simulink model "IEEE9_case"  (R2024b)
settings: Solver=FixedStepAuto  StartTime=0  StopTime=5  FixedStep=1e-7  RelTol=1e-3
values from neighbouring files (symbols this model uses):
  SG_D_1_D = 0.01056    [IEEE9_case_parameters.m]    (also in case1_parameters.m; case2_parameters.m; case3_parameters.m; case4_parameters.m)
  SG_D_1_EnableSaturation = 0    [IEEE9_case_parameters.m]    (also in case1_parameters.m; case2_parameters.m; case3_parameters.m; case4_parameters.m)
  SG_D_1_f0 = 60    [IEEE9_case_parameters.m]    (also in case1_parameters.m; case2_parameters.m; case3_parameters.m; case4_parameters.m)
  SG_D_1_H = 7.5    [IEEE9_case_parameters.m]    (also in case1_parameters.m; case2_parameters.m; case3_parameters.m; case4_parameters.m)
  SG_D_1_K_A = 20    [IEEE9_case_parameters.m]    (also in case1_parameters.m; case2_parameters.m; case3_parameters.m; case4_parameters.m)
  SG_D_1_K_E = 1.000000e+1    (= 10)    [IEEE9_case_parameters.m]    (also in case1_parameters.m; case2_parameters.m; case3_parameters.m; case4_parameters.m)
  SG_D_1_K_F = 2.363    [IEEE9_case_parameters.m]    (also in case1_parameters.m; case2_parameters.m; case3_parameters.m; case4_parameters.m)
  SG_D_1_K_s = 0.5    [IEEE9_case_parameters.m]    (also in case1_parameters.m = 5; case2_parameters.m = 5; case3_parameters.m = 5; case4_parameters.m = 5)
  SG_D_1_R_a = 0.001088    [IEEE9_case_parameters.m]    (also in case1_parameters.m; case2_parameters.m; case3_parameters.m; case4_parameters.m)
  SG_D_1_S_A = 1    [IEEE9_case_parameters.m]    (also in case1_parameters.m; case2_parameters.m; case3_parameters.m; case4_parameters.m)
  SG_D_1_S_B = 0.103    [IEEE9_case_parameters.m]    (also in case1_parameters.m; case2_parameters.m; case3_parameters.m; case4_parameters.m)
  SG_D_1_S_N = 10.659857    [IEEE9_case_parameters.m]    (also in case1_parameters.m; case2_parameters.m; case3_parameters.m; case4_parameters.m)
  SG_D_1_SpeedPara = 200    [IEEE9_case_parameters.m]    (also in case1_parameters.m; case2_parameters.m; case3_parameters.m; case4_parameters.m)
  SG_D_1_T_0 = 0.720173    [IEEE9_case_parameters.m]    (also in case1_parameters.m = 0.755522; case2_parameters.m = 0.808931; case3_parameters.m = 0.869402; case4_parameters.m = 0.729316)
  SG_D_1_T_1 = 0.3    [IEEE9_case_parameters.m]    (also in case1_parameters.m; case2_parameters.m; case3_parameters.m; case4_parameters.m)
  SG_D_1_T_2 = 0.05    [IEEE9_case_parameters.m]    (also in case1_parameters.m; case2_parameters.m; case3_parameters.m; case4_parameters.m)
  SG_D_1_T_3 = 0.02    [IEEE9_case_parameters.m]    (also in case1_parameters.m; case2_parameters.m; case3_parameters.m; case4_parameters.m)
  SG_D_1_T_4 = 0.005    [IEEE9_case_parameters.m]    (also in case1_parameters.m; case2_parameters.m; case3_parameters.m; case4_parameters.m)
  SG_D_1_T_A = 0.02    [IEEE9_case_parameters.m]    (also in case1_parameters.m; case2_parameters.m; case3_parameters.m; case4_parameters.m)
  SG_D_1_T_dd = 8.000000e+0    (= 8)    [IEEE9_case_parameters.m]    (also in case1_parameters.m; case2_parameters.m; case3_parameters.m; case4_parameters.m)
  SG_D_1_T_ddd = 0.04    [IEEE9_case_parameters.m]    (also in case1_parameters.m; case2_parameters.m; case3_parameters.m; case4_parameters.m)
  SG_D_1_T_E = 0.314    [IEEE9_case_parameters.m]    (also in case1_parameters.m; case2_parameters.m; case3_parameters.m; case4_parameters.m)
  SG_D_1_T_F = 0.35    [IEEE9_case_parameters.m]    (also in case1_parameters.m; case2_parameters.m; case3_parameters.m; case4_parameters.m)
  SG_D_1_T_qd = 0.8    [IEEE9_case_parameters.m]    (also in case1_parameters.m; case2_parameters.m; case3_parameters.m; case4_parameters.m)
  SG_D_1_T_qdd = 0.02    [IEEE9_case_parameters.m]    (also in case1_parameters.m; case2_parameters.m; case3_parameters.m; case4_parameters.m)
  SG_D_1_T_speed = 0.1    [IEEE9_case_parameters.m]    (also in case1_parameters.m = 200; case2_parameters.m = 200; case3_parameters.m = 200; case4_parameters.m = 200)
  SG_D_1_T_w = 0.5    [IEEE9_case_parameters.m]    (also in case1_parameters.m; case2_parameters.m; case3_parameters.m; case4_parameters.m)
  SG_D_1_V_ref = 1.990276    [IEEE9_case_parameters.m]    (also in case1_parameters.m = 2.042296; case2_parameters.m = 2.051388; case3_parameters.m = 2.089584; case4_parameters.m = 2.01845)
  SG_D_1_w_ref = 376.991118    [IEEE9_case_parameters.m]    (also in case1_parameters.m; case2_parameters.m; case3_parameters.m; case4_parameters.m)
  SG_D_1_wb = 6.000000e+1    (= 60)    [IEEE9_case_parameters.m]    (also in case1_parameters.m; case2_parameters.m; case3_parameters.m; case4_parameters.m)
  SG_D_1_x_d = 1.9    [IEEE9_case_parameters.m]    (also in case1_parameters.m; case2_parameters.m; case3_parameters.m; case4_parameters.m)
  SG_D_1_x_dd = 0.302    [IEEE9_case_parameters.m]    (also in case1_parameters.m; case2_parameters.m; case3_parameters.m; case4_parameters.m)
  SG_D_1_x_ddd = 0.204    [IEEE9_case_parameters.m]    (also in case1_parameters.m; case2_parameters.m; case3_parameters.m; case4_parameters.m)
  SG_D_1_x_l = 0.05    [IEEE9_case_parameters.m]    (also in case1_parameters.m; case2_parameters.m; case3_parameters.m; case4_parameters.m)
  SG_D_1_x_q = 1.3    [IEEE9_case_parameters.m]    (also in case1_parameters.m; case2_parameters.m; case3_parameters.m; case4_parameters.m)
  SG_D_1_x_qd = 0.5    [IEEE9_case_parameters.m]    (also in case1_parameters.m; case2_parameters.m; case3_parameters.m; case4_parameters.m)
  SG_D_1_x_qdd = 0.3    [IEEE9_case_parameters.m]    (also in case1_parameters.m; case2_parameters.m; case3_parameters.m; case4_parameters.m)
  SG_D_2_D = 0.02    [IEEE9_case_parameters.m]    (also in case1_parameters.m; case2_parameters.m; case3_parameters.m; case4_parameters.m)
  SG_D_2_EnableSaturation = 0    [IEEE9_case_parameters.m]    (also in case1_parameters.m; case2_parameters.m; case3_parameters.m; case4_parameters.m)
  SG_D_2_f0 = 60    [IEEE9_case_parameters.m]    (also in case1_parameters.m; case2_parameters.m; case3_parameters.m; case4_parameters.m)
  SG_D_2_H = 8.000000e+0    (= 8)    [IEEE9_case_parameters.m]    (also in case1_parameters.m; case2_parameters.m; case3_parameters.m; case4_parameters.m)
  SG_D_2_K_A = 20    [IEEE9_case_parameters.m]    (also in case1_parameters.m; case2_parameters.m; case3_parameters.m; case4_parameters.m)
  SG_D_2_K_E = 1.000000e+1    (= 10)    [IEEE9_case_parameters.m]    (also in case1_parameters.m; case2_parameters.m; case3_parameters.m; case4_parameters.m)
  SG_D_2_K_F = 2.363    [IEEE9_case_parameters.m]    (also in case1_parameters.m; case2_parameters.m; case3_parameters.m; case4_parameters.m)
  SG_D_2_K_s = 0.5    [IEEE9_case_parameters.m]    (also in case1_parameters.m = 4; case2_parameters.m = 4; case3_parameters.m = 4; case4_parameters.m = 4)
  SG_D_2_R_a = 0.001088    [IEEE9_case_parameters.m]    (also in case1_parameters.m; case2_parameters.m; case3_parameters.m; case4_parameters.m)
  SG_D_2_S_A = 1    [IEEE9_case_parameters.m]    (also in case1_parameters.m; case2_parameters.m; case3_parameters.m; case4_parameters.m)
  SG_D_2_S_B = 0.103    [IEEE9_case_parameters.m]    (also in case1_parameters.m; case2_parameters.m; case3_parameters.m; case4_parameters.m)
  SG_D_2_S_N = 10.659857    [IEEE9_case_parameters.m]    (also in case1_parameters.m; case2_parameters.m; case3_parameters.m; case4_parameters.m)
  SG_D_2_SpeedPara = 200    [IEEE9_case_parameters.m]    (also in case1_parameters.m; case2_parameters.m; case3_parameters.m; case4_parameters.m)
  SG_D_2_T_0 = 1.632913    [IEEE9_case_parameters.m]    (also in case1_parameters.m = 1.632925; case2_parameters.m = 1.632915; case3_parameters.m = 1.632914; case4_parameters.m = 1.632927)
  SG_D_2_T_1 = 0.2    [IEEE9_case_parameters.m]    (also in case1_parameters.m; case2_parameters.m; case3_parameters.m; case4_parameters.m)
  SG_D_2_T_2 = 0.05    [IEEE9_case_parameters.m]    (also in case1_parameters.m; case2_parameters.m; case3_parameters.m; case4_parameters.m)
  SG_D_2_T_3 = 0.02    [IEEE9_case_parameters.m]    (also in case1_parameters.m; case2_parameters.m; case3_parameters.m; case4_parameters.m)
  SG_D_2_T_4 = 0.005    [IEEE9_case_parameters.m]    (also in case1_parameters.m; case2_parameters.m; case3_parameters.m; case4_parameters.m)
  SG_D_2_T_A = 0.02    [IEEE9_case_parameters.m]    (also in case1_parameters.m; case2_parameters.m; case3_parameters.m; case4_parameters.m)
  SG_D_2_T_dd = 7.9    [IEEE9_case_parameters.m]    (also in case1_parameters.m; case2_parameters.m; case3_parameters.m; case4_parameters.m)
  SG_D_2_T_ddd = 0.04    [IEEE9_case_parameters.m]    (also in case1_parameters.m; case2_parameters.m; case3_parameters.m; case4_parameters.m)
  SG_D_2_T_E = 0.314    [IEEE9_case_parameters.m]    (also in case1_parameters.m; case2_parameters.m; case3_parameters.m; case4_parameters.m)
  SG_D_2_T_F = 0.35    [IEEE9_case_parameters.m]    (also in case1_parameters.m; case2_parameters.m; case3_parameters.m; case4_parameters.m)
  SG_D_2_T_qd = 0.8    [IEEE9_case_parameters.m]    (also in case1_parameters.m; case2_parameters.m; case3_parameters.m; case4_parameters.m)
  SG_D_2_T_qdd = 0.015    [IEEE9_case_parameters.m]    (also in case1_parameters.m; case2_parameters.m; case3_parameters.m; case4_parameters.m)
  SG_D_2_T_speed = 0.1    [IEEE9_case_parameters.m]    (also in case1_parameters.m = 150; case2_parameters.m = 150; case3_parameters.m = 150; case4_parameters.m = 150)
  SG_D_2_T_w = 0.35    [IEEE9_case_parameters.m]    (also in case1_parameters.m; case2_parameters.m; case3_parameters.m; case4_parameters.m)
  SG_D_2_V_ref = 2.58547    [IEEE9_case_parameters.m]    (also in case1_parameters.m = 2.597896; case2_parameters.m = 2.587136; case3_parameters.m = 2.586042; case4_parameters.m = 2.599679)
  SG_D_2_w_ref = 376.991118    [IEEE9_case_parameters.m]    (also in case1_parameters.m; case2_parameters.m; case3_parameters.m; case4_parameters.m)
  SG_D_2_wb = 6.000000e+1    (= 60)    [IEEE9_case_parameters.m]    (also in case1_parameters.m; case2_parameters.m; case3_parameters.m; case4_parameters.m)
  SG_D_2_x_d = 1.8    [IEEE9_case_parameters.m]    (also in case1_parameters.m; case2_parameters.m; case3_parameters.m; case4_parameters.m)
  SG_D_2_x_dd = 0.302    [IEEE9_case_parameters.m]    (also in case1_parameters.m; case2_parameters.m; case3_parameters.m; case4_parameters.m)
  SG_D_2_x_ddd = 0.204    [IEEE9_case_parameters.m]    (also in case1_parameters.m; case2_parameters.m; case3_parameters.m; case4_parameters.m)
  SG_D_2_x_l = 0.05    [IEEE9_case_parameters.m]    (also in case1_parameters.m; case2_parameters.m; case3_parameters.m; case4_parameters.m)
  SG_D_2_x_q = 1.25    [IEEE9_case_parameters.m]    (also in case1_parameters.m; case2_parameters.m; case3_parameters.m; case4_parameters.m)
  SG_D_2_x_qd = 0.5    [IEEE9_case_parameters.m]    (also in case1_parameters.m; case2_parameters.m; case3_parameters.m; case4_parameters.m)
  SG_D_2_x_qdd = 0.3    [IEEE9_case_parameters.m]    (also in case1_parameters.m; case2_parameters.m; case3_parameters.m; case4_parameters.m)
  SG_D_3_D = 0.02    [IEEE9_case_parameters.m]    (also in case1_parameters.m; case2_parameters.m; case3_parameters.m; case4_parameters.m)
  SG_D_3_EnableSaturation = 0    [IEEE9_case_parameters.m]    (also in case1_parameters.m; case2_parameters.m; case3_parameters.m; case4_parameters.m)
  SG_D_3_f0 = 60    [IEEE9_case_parameters.m]    (also in case1_parameters.m; case2_parameters.m; case3_parameters.m; case4_parameters.m)
  SG_D_3_H = 7.7    [IEEE9_case_parameters.m]    (also in case1_parameters.m; case2_parameters.m; case3_parameters.m; case4_parameters.m)
  SG_D_3_K_A = 20    [IEEE9_case_parameters.m]    (also in case1_parameters.m; case2_parameters.m; case3_parameters.m; case4_parameters.m)
  SG_D_3_K_E = 1.000000e+1    (= 10)    [IEEE9_case_parameters.m]    (also in case1_parameters.m; case2_parameters.m; case3_parameters.m; case4_parameters.m)
  SG_D_3_K_F = 2.363    [IEEE9_case_parameters.m]    (also in case1_parameters.m; case2_parameters.m; case3_parameters.m; case4_parameters.m)
  SG_D_3_K_s = 0.2    [IEEE9_case_parameters.m]    (also in case1_parameters.m = 2; case2_parameters.m = 2; case3_parameters.m = 2; case4_parameters.m = 2)
  SG_D_3_R_a = 0.001088    [IEEE9_case_parameters.m]    (also in case1_parameters.m; case2_parameters.m; case3_parameters.m; case4_parameters.m)
  SG_D_3_S_A = 1    [IEEE9_case_parameters.m]    (also in case1_parameters.m; case2_parameters.m; case3_parameters.m; case4_parameters.m)
  SG_D_3_S_B = 0.103    [IEEE9_case_parameters.m]    (also in case1_parameters.m; case2_parameters.m; case3_parameters.m; case4_parameters.m)
  SG_D_3_S_N = 10.659857    [IEEE9_case_parameters.m]    (also in case1_parameters.m; case2_parameters.m; case3_parameters.m; case4_parameters.m)
  SG_D_3_SpeedPara = 200    [IEEE9_case_parameters.m]    (also in case1_parameters.m; case2_parameters.m; case3_parameters.m; case4_parameters.m)
  SG_D_3_T_0 = 0.850788    [IEEE9_case_parameters.m]    (also in case1_parameters.m = 0.850786; case2_parameters.m = 0.850787; case3_parameters.m; case4_parameters.m = 0.850786)
  SG_D_3_T_1 = 0.2    [IEEE9_case_parameters.m]    (also in case1_parameters.m; case2_parameters.m; case3_parameters.m; case4_parameters.m)
  SG_D_3_T_2 = 0.05    [IEEE9_case_parameters.m]    (also in case1_parameters.m; case2_parameters.m; case3_parameters.m; case4_parameters.m)
  SG_D_3_T_3 = 0.02    [IEEE9_case_parameters.m]    (also in case1_parameters.m; case2_parameters.m; case3_parameters.m; case4_parameters.m)
  SG_D_3_T_4 = 0.005    [IEEE9_case_parameters.m]    (also in case1_parameters.m; case2_parameters.m; case3_parameters.m; case4_parameters.m)
  SG_D_3_T_A = 0.02    [IEEE9_case_parameters.m]    (also in case1_parameters.m; case2_parameters.m; case3_parameters.m; case4_parameters.m)
  SG_D_3_T_dd = 8.1    [IEEE9_case_parameters.m]    (also in case1_parameters.m; case2_parameters.m; case3_parameters.m; case4_parameters.m)
  SG_D_3_T_ddd = 0.04    [IEEE9_case_parameters.m]    (also in case1_parameters.m; case2_parameters.m; case3_parameters.m; case4_parameters.m)
  SG_D_3_T_E = 0.314    [IEEE9_case_parameters.m]    (also in case1_parameters.m; case2_parameters.m; case3_parameters.m; case4_parameters.m)
  SG_D_3_T_F = 0.35    [IEEE9_case_parameters.m]    (also in case1_parameters.m; case2_parameters.m; case3_parameters.m; case4_parameters.m)
  SG_D_3_T_qd = 0.8    [IEEE9_case_parameters.m]    (also in case1_parameters.m; case2_parameters.m; case3_parameters.m; case4_parameters.m)
  SG_D_3_T_qdd = 0.015    [IEEE9_case_parameters.m]    (also in case1_parameters.m; case2_parameters.m; case3_parameters.m; case4_parameters.m)
  SG_D_3_T_speed = 0.1    [IEEE9_case_parameters.m]    (also in case1_parameters.m = 180; case2_parameters.m = 180; case3_parameters.m = 180; case4_parameters.m = 180)
  SG_D_3_T_w = 0.4    [IEEE9_case_parameters.m]    (also in case1_parameters.m; case2_parameters.m; case3_parameters.m; case4_parameters.m)
  SG_D_3_V_ref = 1.892727    [IEEE9_case_parameters.m]    (also in case1_parameters.m = 1.906439; case2_parameters.m = 1.895535; case3_parameters.m = 1.892105; case4_parameters.m = 1.906598)
  SG_D_3_w_ref = 376.991118    [IEEE9_case_parameters.m]    (also in case1_parameters.m; case2_parameters.m; case3_parameters.m; case4_parameters.m)
  SG_D_3_wb = 6.000000e+1    (= 60)    [IEEE9_case_parameters.m]    (also in case1_parameters.m; case2_parameters.m; case3_parameters.m; case4_parameters.m)
  SG_D_3_x_d = 1.85    [IEEE9_case_parameters.m]    (also in case1_parameters.m; case2_parameters.m; case3_parameters.m; case4_parameters.m)
  SG_D_3_x_dd = 0.302    [IEEE9_case_parameters.m]    (also in case1_parameters.m; case2_parameters.m; case3_parameters.m; case4_parameters.m)
  SG_D_3_x_ddd = 0.204    [IEEE9_case_parameters.m]    (also in case1_parameters.m; case2_parameters.m; case3_parameters.m; case4_parameters.m)
  SG_D_3_x_l = 0.05    [IEEE9_case_parameters.m]    (also in case1_parameters.m; case2_parameters.m; case3_parameters.m; case4_parameters.m)
  SG_D_3_x_q = 1.2    [IEEE9_case_parameters.m]    (also in case1_parameters.m; case2_parameters.m; case3_parameters.m; case4_parameters.m)
  SG_D_3_x_qd = 0.5    [IEEE9_case_parameters.m]    (also in case1_parameters.m; case2_parameters.m; case3_parameters.m; case4_parameters.m)
  SG_D_3_x_qdd = 0.3    [IEEE9_case_parameters.m]    (also in case1_parameters.m; case2_parameters.m; case3_parameters.m; case4_parameters.m)
(part 9 of 12)

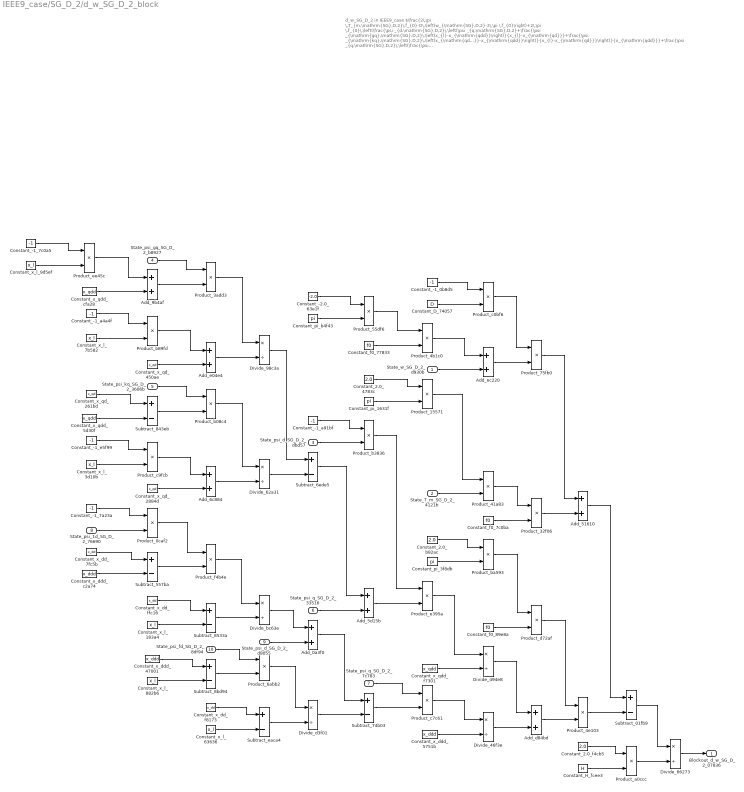
== system IEEE9_case/SG_D_2/d_w_SG_D_2_block ==
  note: d_w_SG_D_2 in IEEE9_case
      | $\frac{2\,\pi \,T_{m,\mathrm{SG},D,2}\,f_{0}-D\,\left(w_{\mathrm{SG},D,2}-2\,\pi \,f_{0}\right)+2\,\pi \,f_{0}\,\left(\frac{\psi _{d,\mathrm{SG},D,2}\,\left(\psi _{q,\mathrm{SG},D,2}+\frac{\psi _{\mathrm{gq},\mathrm{SG},D,2}\,\left(x_{l}-x_{\mathrm{qdd}}\right)}{x_{l}-x_{\mathrm{qd}}}+\frac{\psi _{\mathrm{kq},\mathrm{SG},D,2}\,\left(x_{\mathrm{qd}}-x_{\mathrm{qdd}}\right)}{x_{l}-x_{\mathrm{qd}}}\right)}{x_{\mathrm{qdd}}}+\frac{\psi _{q,\mathrm{SG},D,2}\,\left(\frac{\psi _{\mathrm{1d},\mathrm{SG},D,2}\,\left(x_{\mathrm{dd}}-x_{\mathrm{ddd}}\right)}{x_{\mathrm{dd}}-x_{l}}-\psi _{d,\mathrm{SG},D,2}+\frac{\psi _{\mathrm{fd},\mathrm{SG},D,2}\,\left(x_{\mathrm{ddd}}-x_{l}\right)}{x_{\mathrm{dd}}-x_{l}}\right)}{x_{\mathrm{ddd}}}\right)}{2\,H}$
      | Automatically generated on 2025-11-01 08:48:58 .
  State_w_SG_D_2_d930b : Inport
  State_T_m_SG_D_2_4121b : Inport  Port=2
  State_psi_d_SG_D_2_dbd57 : Inport  Port=3
  State_psi_gq_SG_D_2_b8927 : Inport  Port=4
  State_psi_kq_SG_D_2_3606b : Inport  Port=5
  State_psi_q_SG_D_2_33516 : Inport  Port=6
  State_psi_q_SG_D_2_7c783 : Inport  Port=7
  State_psi_1d_SG_D_2_76690 : Inport  Port=8
  State_psi_d_SG_D_2_d8055 : Inport  Port=9
  State_psi_fd_SG_D_2_8df94 : Inport  Port=10
  Add_0a3f0 : Sum
  Add_51610 : Sum
  Add_5d15b : Sum
  Add_6c884 : Sum
  Add_9b4af : Sum
  Add_d84bd : Sum
  Add_e04e4 : Sum
  Add_ec220 : Sum
  Constant_-1_0b8d5 : Constant  Value=-1
  Constant_-1_7a23a : Constant  Value=-1
  Constant_-1_7c0a5 : Constant  Value=-1
  Constant_-1_a4a4f : Constant  Value=-1
  Constant_-1_a91bf : Constant  Value=-1
  Constant_-1_e5f99 : Constant  Value=-1
  Constant_-2.0_63e1f : Constant  Value=-2.0
  Constant_2.0_4783c : Constant  Value=2.0
  Constant_2.0_b82ac : Constant  Value=2.0
  Constant_2.0_f4cb5 : Constant  Value=2.0
  Constant_D_74057 : Constant  Value=D
  Constant_H_fcee3 : Constant  Value=H
  Constant_f0_77833 : Constant  Value=f0
  Constant_f0_7c0ba : Constant  Value=f0
  Constant_f0_89e8a : Constant  Value=f0
  Constant_pi_1631f : Constant  Value=pi
  Constant_pi_3f8db : Constant  Value=pi
  Constant_pi_b4f43 : Constant  Value=pi
  Constant_x_dd_7fc5b : Constant  Value=x_dd
  Constant_x_dd_f8173 : Constant  Value=x_dd
  Constant_x_dd_ffc16 : Constant  Value=x_dd
  Constant_x_ddd_47001 : Constant  Value=x_ddd
  Constant_x_ddd_5751b : Constant  Value=x_ddd
  Constant_x_ddd_c2a74 : Constant  Value=x_ddd
  Constant_x_l_183a4 : Constant  Value=x_l
  Constant_x_l_3d10b : Constant  Value=x_l
  Constant_x_l_63636 : Constant  Value=x_l
  Constant_x_l_7b582 : Constant  Value=x_l
  Constant_x_l_882b6 : Constant  Value=x_l
  Constant_x_l_9d5ef : Constant  Value=x_l
  Constant_x_qd_261bd : Constant  Value=x_qd
  Constant_x_qd_2884d : Constant  Value=x_qd
  Constant_x_qd_450ae : Constant  Value=x_qd
  Constant_x_qdd_5d30f : Constant  Value=x_qdd
  Constant_x_qdd_cfa28 : Constant  Value=x_qdd
  Constant_x_qdd_f7301 : Constant  Value=x_qdd
  Divide_46f3e : Product  Inputs=*/
  Divide_494e8 : Product  Inputs=*/
  Divide_62a31 : Product  Inputs=*/
  Divide_66273 : Product  Inputs=*/
  Divide_98c3a : Product  Inputs=*/
  Divide_bc63e : Product  Inputs=*/
  Divide_d3f01 : Product  Inputs=*/
  Product_0caf2 : Product
  Product_15571 : Product
  Product_32f06 : Product
  Product_3add3 : Product
  Product_41a83 : Product
  Product_4b1c0 : Product
  Product_4e103 : Product
  Product_55df6 : Product
  Product_6abb2 : Product
  Product_75fb0 : Product
  Product_a0ccc : Product
  Product_b08c4 : Product
  Product_b3836 : Product
  Product_b89fd : Product
  Product_ba593 : Product
  Product_c0bf6 : Product
  Product_c7c61 : Product
  Product_c9fcb : Product
  Product_d72af : Product
  Product_e395a : Product
  Product_ee45c : Product
  Product_f4b4e : Product
  Subtract_01fb9 : Sum  Inputs=+-
  Subtract_557ba : Sum  Inputs=+-
  Subtract_6ede5 : Sum  Inputs=+-
  Subtract_74b03 : Sum  Inputs=+-
  Subtract_843eb : Sum  Inputs=+-
  Subtract_8533a : Sum  Inputs=+-
  Subtract_8bd94 : Sum  Inputs=+-
  Subtract_eaca4 : Sum  Inputs=+-
  Blockout_d_w_SG_D_2_07836 : Outport
  wires:
  Constant_x_qd_261bd/1 -> Subtract_843eb/1
  Constant_-1_e5f99/1 -> Product_c9fcb/1
  Constant_-1_7c0a5/1 -> Product_ee45c/1
  Constant_x_qdd_5d30f/1 -> Subtract_843eb/2
  Subtract_eaca4/1 -> Divide_d3f01/2
  Constant_x_l_3d10b/1 -> Product_c9fcb/2
  Constant_x_l_9d5ef/1 -> Product_ee45c/2
  Product_c9fcb/1 -> Add_6c884/1
  Product_ee45c/1 -> Add_9b4af/1
  Constant_x_l_183a4/1 -> Subtract_8533a/2
  Constant_x_l_7b582/1 -> Product_b89fd/2
  Constant_x_ddd_5751b/1 -> Divide_46f3e/2
  Subtract_8bd94/1 -> Product_6abb2/2
  Constant_x_qd_2884d/1 -> Add_6c884/2
  Constant_x_qdd_cfa28/1 -> Add_9b4af/2
  Constant_-1_a4a4f/1 -> Product_b89fd/1
  State_psi_d_SG_D_2_dbd57/1 -> Product_b3836/2
  Constant_-1_7a23a/1 -> Product_0caf2/1
  State_w_SG_D_2_d930b/1 -> Add_ec220/2
  Product_b89fd/1 -> Add_e04e4/1
  State_psi_1d_SG_D_2_76690/1 -> Product_0caf2/2
  Constant_x_dd_7fc5b/1 -> Subtract_557ba/1
  Divide_98c3a/1 -> Subtract_6ede5/1
  Subtract_843eb/1 -> Product_b08c4/2
  Constant_x_ddd_c2a74/1 -> Subtract_557ba/2
  State_psi_gq_SG_D_2_b8927/1 -> Product_3add3/1
  Add_6c884/1 -> Divide_62a31/2
  State_psi_d_SG_D_2_d8055/1 -> Add_0a3f0/2
  Add_9b4af/1 -> Product_3add3/2
  Constant_x_qd_450ae/1 -> Add_e04e4/2
  State_psi_kq_SG_D_2_3606b/1 -> Product_b08c4/1
  Product_0caf2/1 -> Product_f4b4e/1
  Subtract_557ba/1 -> Product_f4b4e/2
  Constant_pi_1631f/1 -> Product_15571/2
  Constant_x_dd_ffc16/1 -> Subtract_8533a/1
  Constant_x_ddd_47001/1 -> Subtract_8bd94/1
  Constant_x_l_882b6/1 -> Subtract_8bd94/2
  Product_3add3/1 -> Divide_98c3a/1
  Add_e04e4/1 -> Divide_98c3a/2
  Add_5d15b/1 -> Product_e395a/2
  Product_b08c4/1 -> Divide_62a31/1
  Constant_pi_b4f43/1 -> Product_55df6/2
  Product_f4b4e/1 -> Divide_bc63e/1
  Subtract_8533a/1 -> Divide_bc63e/2
  State_psi_fd_SG_D_2_8df94/1 -> Product_6abb2/1
  Divide_bc63e/1 -> Add_0a3f0/1
  Constant_x_dd_f8173/1 -> Subtract_eaca4/1
  Constant_x_l_63636/1 -> Subtract_eaca4/2
  Divide_62a31/1 -> Subtract_6ede5/2
  Product_6abb2/1 -> Divide_d3f01/1
  Constant_-1_a91bf/1 -> Product_b3836/1
  Constant_-2.0_63e1f/1 -> Product_55df6/1
  Subtract_6ede5/1 -> Add_5d15b/1
  Subtract_74b03/1 -> Product_c7c61/2
  State_psi_q_SG_D_2_33516/1 -> Add_5d15b/2
  Constant_D_74057/1 -> Product_c0bf6/2
  Add_0a3f0/1 -> Subtract_74b03/1
  Divide_d3f01/1 -> Subtract_74b03/2
  Product_55df6/1 -> Product_4b1c0/1
  Constant_f0_77833/1 -> Product_4b1c0/2
  Constant_2.0_4783c/1 -> Product_15571/1
  Product_b3836/1 -> Product_e395a/1
  State_psi_q_SG_D_2_7c783/1 -> Product_c7c61/1
  Constant_-1_0b8d5/1 -> Product_c0bf6/1
  Product_4b1c0/1 -> Add_ec220/1
  Product_15571/1 -> Product_41a83/1
  State_T_m_SG_D_2_4121b/1 -> Product_41a83/2
  Constant_2.0_b82ac/1 -> Product_ba593/1
  Constant_pi_3f8db/1 -> Product_ba593/2
  Product_e395a/1 -> Divide_494e8/1
  Constant_x_qdd_f7301/1 -> Divide_494e8/2
  Product_c7c61/1 -> Divide_46f3e/1
  Product_c0bf6/1 -> Product_75fb0/1
  Add_ec220/1 -> Product_75fb0/2
  Product_41a83/1 -> Product_32f06/1
  Constant_f0_7c0ba/1 -> Product_32f06/2
  Product_ba593/1 -> Product_d72af/1
  Constant_f0_89e8a/1 -> Product_d72af/2
  Divide_494e8/1 -> Add_d84bd/1
  Divide_46f3e/1 -> Add_d84bd/2
  Product_75fb0/1 -> Add_51610/1
  Product_32f06/1 -> Add_51610/2
  Product_d72af/1 -> Product_4e103/1
  Add_d84bd/1 -> Product_4e103/2
  Add_51610/1 -> Subtract_01fb9/1
  Product_4e103/1 -> Subtract_01fb9/2
  Constant_2.0_f4cb5/1 -> Product_a0ccc/1
  Constant_H_fcee3/1 -> Product_a0ccc/2
  Subtract_01fb9/1 -> Divide_66273/1
  Product_a0ccc/1 -> Divide_66273/2
  Divide_66273/1 -> Blockout_d_w_SG_D_2_07836/1

== system IEEE9_case/SG_D_2/i_d_SG_D_2_block ==
  note: i_d_SG_D_2 in IEEE9_case
      | $\frac{\sin\left(\theta _{\mathrm{SG},D,2}\right)\,\left(\frac{\psi _{\mathrm{1d},\mathrm{SG},D,2}\,\left(x_{\mathrm{dd}}-x_{\mathrm{ddd}}\right)}{x_{\mathrm{dd}}-x_{l}}-\psi _{d,\mathrm{SG},D,2}+\frac{\psi _{\mathrm{fd},\mathrm{SG},D,2}\,\left(x_{\mathrm{ddd}}-x_{l}\right)}{x_{\mathrm{dd}}-x_{l}}\right)}{x_{\mathrm{ddd}}}-\frac{\cos\left(\theta _{\mathrm{SG},D,2}\right)\,\left(\psi _{q,\mathrm{SG},D,2}+\frac{\psi _{\mathrm{gq},\mathrm{SG},D,2}\,\left(x_{l}-x_{\mathrm{qdd}}\right)}{x_{l}-x_{\mathrm{qd}}}+\frac{\psi _{\mathrm{kq},\mathrm{SG},D,2}\,\left(x_{\mathrm{qd}}-x_{\mathrm{qdd}}\right)}{x_{l}-x_{\mathrm{qd}}}\right)}{x_{\mathrm{qdd}}}$
      | Automatically generated on 2025-11-01 08:49:20 .
  State_psi_gq_SG_D_2_c758c : Inport
  State_psi_kq_SG_D_2_22efa : Inport  Port=2
  State_psi_q_SG_D_2_90cca : Inport  Port=3
  State_theta_SG_D_2_b69be : Inport  Port=4
  State_psi_1d_SG_D_2_5d51d : Inport  Port=5
  State_psi_d_SG_D_2_f7721 : Inport  Port=6
  State_psi_fd_SG_D_2_83be3 : Inport  Port=7
  State_theta_SG_D_2_1b926 : Inport  Port=8
  Add_16b33 : Sum
  Add_2a93c : Sum
  Add_7d69f : Sum
  Add_a40ae : Sum
  Add_b9970 : Sum
  Constant_-1_8a7ae : Constant  Value=-1
  Constant_-1_a0e83 : Constant  Value=-1
  Constant_-1_cca40 : Constant  Value=-1
  Constant_-1_e0227 : Constant  Value=-1
  Constant_-1_f6edc : Constant  Value=-1
  Constant_x_dd_486e3 : Constant  Value=x_dd
  Constant_x_dd_9e9c9 : Constant  Value=x_dd
  Constant_x_dd_f4509 : Constant  Value=x_dd
  Constant_x_ddd_62481 : Constant  Value=x_ddd
  Constant_x_ddd_8778a : Constant  Value=x_ddd
  Constant_x_ddd_cb7be : Constant  Value=x_ddd
  Constant_x_l_225f2 : Constant  Value=x_l
  Constant_x_l_3670c : Constant  Value=x_l
  Constant_x_l_5d8a7 : Constant  Value=x_l
  Constant_x_l_7740d : Constant  Value=x_l
  Constant_x_l_c677c : Constant  Value=x_l
  Constant_x_l_cd01c : Constant  Value=x_l
  Constant_x_qd_0d99f : Constant  Value=x_qd
  Constant_x_qd_c1993 : Constant  Value=x_qd
  Constant_x_qd_dd2b1 : Constant  Value=x_qd
  Constant_x_qdd_63b5a : Constant  Value=x_qdd
  Constant_x_qdd_7c187 : Constant  Value=x_qdd
  Constant_x_qdd_ddcc5 : Constant  Value=x_qdd
  Divide_1d12e : Product  Inputs=*/
  Divide_4dcec : Product  Inputs=*/
  Divide_68914 : Product  Inputs=*/
  Divide_e1176 : Product  Inputs=*/
  Divide_e527e : Product  Inputs=*/
  Divide_ec32b : Product  Inputs=*/
  MathFunc_cos_7f3e3 : Trigonometry  Operator=cos
  MathFunc_sin_ceb21 : Trigonometry
  Product_32228 : Product
  Product_4e613 : Product
  Product_50eb5 : Product
  Product_69a70 : Product
  Product_80f0d : Product
  Product_94158 : Product
  Product_cbd1a : Product
  Product_d4211 : Product
  Product_f1ae8 : Product
  Product_f7996 : Product
  Product_f9eb1 : Product
  Subtract_1405e : Sum  Inputs=+-
  Subtract_2754a : Sum  Inputs=+-
  Subtract_4e6d5 : Sum  Inputs=+-
  Subtract_55bd6 : Sum  Inputs=+-
  Subtract_b72de : Sum  Inputs=+-
  Subtract_c13ca : Sum  Inputs=+-
  Subtract_d6086 : Sum  Inputs=+-
  Subtract_f8817 : Sum  Inputs=+-
  Blockout_i_d_SG_D_2_05ed7 : Outport
  wires:
  Constant_x_ddd_62481/1 -> Subtract_55bd6/1
  Constant_x_qd_dd2b1/1 -> Subtract_1405e/1
  Constant_-1_cca40/1 -> Product_cbd1a/1
  Constant_-1_f6edc/1 -> Product_94158/1
  Subtract_2754a/1 -> Blockout_i_d_SG_D_2_05ed7/1
  Constant_x_qdd_ddcc5/1 -> Subtract_1405e/2
  Constant_x_l_cd01c/1 -> Product_cbd1a/2
  Constant_x_l_5d8a7/1 -> Product_94158/2
  Product_cbd1a/1 -> Add_7d69f/1
  Product_94158/1 -> Add_b9970/1
  Constant_x_l_c677c/1 -> Product_4e613/2
  Constant_x_qd_c1993/1 -> Add_7d69f/2
  Constant_x_qdd_63b5a/1 -> Add_b9970/2
  Constant_x_qdd_7c187/1 -> Divide_e527e/2
  MathFunc_cos_7f3e3/1 -> Product_f7996/2
  Constant_-1_e0227/1 -> Product_4e613/1
  State_psi_gq_SG_D_2_c758c/1 -> Product_80f0d/1
  Subtract_55bd6/1 -> Product_f1ae8/2
  Product_f9eb1/1 -> Product_d4211/1
  Add_7d69f/1 -> Divide_4dcec/2
  Add_b9970/1 -> Product_80f0d/2
  Product_f1ae8/1 -> Divide_e1176/1
  Product_4e613/1 -> Add_16b33/1
  Constant_x_qd_0d99f/1 -> Add_16b33/2
  State_theta_SG_D_2_1b926/1 -> MathFunc_sin_ceb21/1
  State_psi_kq_SG_D_2_22efa/1 -> Product_69a70/1
  Add_a40ae/1 -> Subtract_4e6d5/1
  Subtract_1405e/1 -> Product_69a70/2
  Product_80f0d/1 -> Divide_ec32b/1
  Constant_-1_a0e83/1 -> Product_f9eb1/1
  State_psi_1d_SG_D_2_5d51d/1 -> Product_f9eb1/2
  State_psi_fd_SG_D_2_83be3/1 -> Product_f1ae8/1
  Constant_x_dd_9e9c9/1 -> Subtract_f8817/1
  Product_d4211/1 -> Divide_68914/1
  Constant_x_ddd_8778a/1 -> Subtract_f8817/2
  Divide_e1176/1 -> Subtract_4e6d5/2
  Add_16b33/1 -> Divide_ec32b/2
  Product_50eb5/1 -> Divide_1d12e/1
  Product_69a70/1 -> Divide_4dcec/1
  Constant_-1_8a7ae/1 -> Product_32228/1
  Subtract_d6086/1 -> Divide_e1176/2
  Subtract_f8817/1 -> Product_d4211/2
  Constant_x_dd_f4509/1 -> Subtract_b72de/1
  Subtract_4e6d5/1 -> Product_50eb5/1
  Constant_x_l_3670c/1 -> Subtract_b72de/2
  Constant_x_l_7740d/1 -> Subtract_55bd6/2
  Divide_ec32b/1 -> Subtract_c13ca/1
  Divide_1d12e/1 -> Subtract_2754a/2
  Divide_4dcec/1 -> Subtract_c13ca/2
  Subtract_b72de/1 -> Divide_68914/2
  Constant_x_dd_486e3/1 -> Subtract_d6086/1
  Divide_e527e/1 -> Subtract_2754a/1
  Constant_x_l_225f2/1 -> Subtract_d6086/2
  Subtract_c13ca/1 -> Add_2a93c/1
  State_psi_q_SG_D_2_90cca/1 -> Add_2a93c/2
  Constant_x_ddd_cb7be/1 -> Divide_1d12e/2
  MathFunc_sin_ceb21/1 -> Product_50eb5/2
  Divide_68914/1 -> Add_a40ae/1
  State_psi_d_SG_D_2_f7721/1 -> Add_a40ae/2
  Add_2a93c/1 -> Product_32228/2
  State_theta_SG_D_2_b69be/1 -> MathFunc_cos_7f3e3/1
  Product_32228/1 -> Product_f7996/1
  Product_f7996/1 -> Divide_e527e/1

== system IEEE9_case/SG_D_2/i_q_SG_D_2_block ==
  note: i_q_SG_D_2 in IEEE9_case
      | $-\frac{\sin\left(\theta _{\mathrm{SG},D,2}\right)\,\left(\psi _{q,\mathrm{SG},D,2}+\frac{\psi _{\mathrm{gq},\mathrm{SG},D,2}\,\left(x_{l}-x_{\mathrm{qdd}}\right)}{x_{l}-x_{\mathrm{qd}}}+\frac{\psi _{\mathrm{kq},\mathrm{SG},D,2}\,\left(x_{\mathrm{qd}}-x_{\mathrm{qdd}}\right)}{x_{l}-x_{\mathrm{qd}}}\right)}{x_{\mathrm{qdd}}}-\frac{\cos\left(\theta _{\mathrm{SG},D,2}\right)\,\left(\frac{\psi _{\mathrm{1d},\mathrm{SG},D,2}\,\left(x_{\mathrm{dd}}-x_{\mathrm{ddd}}\right)}{x_{\mathrm{dd}}-x_{l}}-\psi _{d,\mathrm{SG},D,2}+\frac{\psi _{\mathrm{fd},\mathrm{SG},D,2}\,\left(x_{\mathrm{ddd}}-x_{l}\right)}{x_{\mathrm{dd}}-x_{l}}\right)}{x_{\mathrm{ddd}}}$
      | Automatically generated on 2025-11-01 08:49:24 .
  State_psi_gq_SG_D_2_0dc4e : Inport
  State_psi_kq_SG_D_2_62e42 : Inport  Port=2
  State_psi_q_SG_D_2_067b4 : Inport  Port=3
  State_theta_SG_D_2_eabbf : Inport  Port=4
  State_psi_1d_SG_D_2_50cf4 : Inport  Port=5
  State_psi_d_SG_D_2_5901a : Inport  Port=6
  State_psi_fd_SG_D_2_97667 : Inport  Port=7
  State_theta_SG_D_2_5175d : Inport  Port=8
  Add_10415 : Sum
  Add_23454 : Sum
  Add_3c0f7 : Sum
  Add_928b7 : Sum
  Add_bff7f : Sum
  Add_e1e39 : Sum
  Constant_-1_02d73 : Constant  Value=-1
  Constant_-1_2b165 : Constant  Value=-1
  Constant_-1_6626f : Constant  Value=-1
  Constant_-1_86c62 : Constant  Value=-1
  Constant_-1_f6aa3 : Constant  Value=-1
  Constant_x_dd_2c0f3 : Constant  Value=x_dd
  Constant_x_dd_7f386 : Constant  Value=x_dd
  Constant_x_dd_fa11b : Constant  Value=x_dd
  Constant_x_ddd_1d224 : Constant  Value=x_ddd
  Constant_x_ddd_44ed5 : Constant  Value=x_ddd
  Constant_x_ddd_cfc8a : Constant  Value=x_ddd
  Constant_x_l_1c58b : Constant  Value=x_l
  Constant_x_l_3b033 : Constant  Value=x_l
  Constant_x_l_8d7a7 : Constant  Value=x_l
  Constant_x_l_a249f : Constant  Value=x_l
  Constant_x_l_b664e : Constant  Value=x_l
  Constant_x_l_facfd : Constant  Value=x_l
  Constant_x_qd_6aaec : Constant  Value=x_qd
  Constant_x_qd_c61d3 : Constant  Value=x_qd
  Constant_x_qd_e0e12 : Constant  Value=x_qd
  Constant_x_qdd_212d8 : Constant  Value=x_qdd
  Constant_x_qdd_dd4ac : Constant  Value=x_qdd
  Constant_x_qdd_e5b79 : Constant  Value=x_qdd
  Divide_13495 : Product  Inputs=*/
  Divide_6505e : Product  Inputs=*/
  Divide_7ba83 : Product  Inputs=*/
  Divide_87098 : Product  Inputs=*/
  Divide_b37c0 : Product  Inputs=*/
  Divide_ccfe0 : Product  Inputs=*/
  MathFunc_cos_c87f3 : Trigonometry  Operator=cos
  MathFunc_sin_5f144 : Trigonometry
  Product_2807a : Product
  Product_31c23 : Product
  Product_38ead : Product
  Product_412fa : Product
  Product_62eea : Product
  Product_83602 : Product
  Product_aec53 : Product
  Product_d52d7 : Product
  Product_e786b : Product
  Product_e9eff : Product
  Product_ed763 : Product
  Subtract_3bd4d : Sum  Inputs=+-
  Subtract_450ad : Sum  Inputs=+-
  Subtract_843d7 : Sum  Inputs=+-
  Subtract_8aebb : Sum  Inputs=+-
  Subtract_9c53a : Sum  Inputs=+-
  Subtract_a071b : Sum  Inputs=+-
  Subtract_a1a72 : Sum  Inputs=+-
  Blockout_i_q_SG_D_2_9bb23 : Outport
  wires:
  MathFunc_sin_5f144/1 -> Product_62eea/2
  Product_83602/1 -> Product_62eea/1
  Constant_-1_6626f/1 -> Product_ed763/1
  Constant_-1_02d73/1 -> Product_e786b/1
  Constant_x_l_b664e/1 -> Product_ed763/2
  Product_ed763/1 -> Add_e1e39/1
  Subtract_a1a72/1 -> Product_2807a/2
  Constant_x_qdd_e5b79/1 -> Subtract_9c53a/2
  Constant_x_qdd_212d8/1 -> Add_e1e39/2
  Add_10415/1 -> Product_83602/2
  Constant_x_l_3b033/1 -> Product_e786b/2
  Constant_x_qd_c61d3/1 -> Subtract_9c53a/1
  Constant_-1_86c62/1 -> Product_e9eff/1
  Constant_x_l_facfd/1 -> Product_e9eff/2
  State_psi_1d_SG_D_2_50cf4/1 -> Product_aec53/2
  State_psi_gq_SG_D_2_0dc4e/1 -> Product_38ead/1
  Add_e1e39/1 -> Product_38ead/2
  Product_e786b/1 -> Add_23454/1
  Divide_13495/1 -> Add_3c0f7/1
  Constant_x_qd_6aaec/1 -> Add_23454/2
  State_psi_kq_SG_D_2_62e42/1 -> Product_31c23/1
  Add_928b7/1 -> Subtract_843d7/1
  Constant_x_ddd_1d224/1 -> Subtract_a1a72/2
  Subtract_9c53a/1 -> Product_31c23/2
  Product_e9eff/1 -> Add_bff7f/1
  Constant_x_qd_e0e12/1 -> Add_bff7f/2
  Constant_-1_2b165/1 -> Product_aec53/1
  Constant_x_l_a249f/1 -> Subtract_8aebb/2
  Constant_x_dd_2c0f3/1 -> Subtract_a1a72/1
  Product_38ead/1 -> Divide_6505e/1
  Divide_87098/1 -> Subtract_843d7/2
  Add_23454/1 -> Divide_6505e/2
  Product_412fa/1 -> Divide_7ba83/1
  Product_31c23/1 -> Divide_ccfe0/1
  Constant_-1_f6aa3/1 -> Product_83602/1
  Product_aec53/1 -> Product_2807a/1
  Add_bff7f/1 -> Divide_ccfe0/2
  Constant_x_dd_fa11b/1 -> Subtract_3bd4d/1
  Subtract_843d7/1 -> Product_412fa/1
  Subtract_a071b/1 -> Product_d52d7/2
  Constant_x_l_1c58b/1 -> Subtract_3bd4d/2
  Constant_x_ddd_44ed5/1 -> Subtract_a071b/1
  Constant_x_l_8d7a7/1 -> Subtract_a071b/2
  Divide_6505e/1 -> Subtract_450ad/1
  Divide_7ba83/1 -> Add_3c0f7/2
  Product_d52d7/1 -> Divide_87098/1
  Divide_ccfe0/1 -> Subtract_450ad/2
  Subtract_8aebb/1 -> Divide_87098/2
  Product_2807a/1 -> Divide_b37c0/1
  Subtract_3bd4d/1 -> Divide_b37c0/2
  Constant_x_qdd_dd4ac/1 -> Divide_13495/2
  State_psi_fd_SG_D_2_97667/1 -> Product_d52d7/1
  Constant_x_dd_7f386/1 -> Subtract_8aebb/1
  Subtract_450ad/1 -> Add_10415/1
  State_psi_q_SG_D_2_067b4/1 -> Add_10415/2
  Constant_x_ddd_cfc8a/1 -> Divide_7ba83/2
  Divide_b37c0/1 -> Add_928b7/1
  State_psi_d_SG_D_2_5901a/1 -> Add_928b7/2
  State_theta_SG_D_2_eabbf/1 -> MathFunc_sin_5f144/1
  State_theta_SG_D_2_5175d/1 -> MathFunc_cos_c87f3/1
  MathFunc_cos_c87f3/1 -> Product_412fa/2
  Product_62eea/1 -> Divide_13495/1
  Add_3c0f7/1 -> Blockout_i_q_SG_D_2_9bb23/1

== system IEEE9_case/SG_D_2/theta_SG_D_2_out_block ==
  note: theta_SG_D_2_out in IEEE9_case
      | $\theta _{\mathrm{SG},D,2}$
      | Automatically generated on 2025-11-01 08:49:30 .
  State_theta_SG_D_2_b5c4c : Inport
  Blockout_theta_SG_D_2_out_8a415 : Outport
  wires:
  State_theta_SG_D_2_b5c4c/1 -> Blockout_theta_SG_D_2_out_8a415/1

== system IEEE9_case/SG_D_2/w_SG_D_2_out_block ==
  note: w_SG_D_2_out in IEEE9_case
      | $w_{\mathrm{SG},D,2}$
      | Automatically generated on 2025-11-01 08:49:29 .
  State_w_SG_D_2_bfe63 : Inport
  Blockout_w_SG_D_2_out_ddf0a : Outport
  wires:
  State_w_SG_D_2_bfe63/1 -> Blockout_w_SG_D_2_out_ddf0a/1

== system IEEE9_case/SG_D_3/T_e_SG_D_3_block ==
  note: T_e_SG_D_3 in IEEE9_case
      | $-\frac{\psi _{d,\mathrm{SG},D,3}\,\left(\psi _{q,\mathrm{SG},D,3}+\frac{\psi _{\mathrm{gq},\mathrm{SG},D,3}\,\left(x_{l}-x_{\mathrm{qdd}}\right)}{x_{l}-x_{\mathrm{qd}}}+\frac{\psi _{\mathrm{kq},\mathrm{SG},D,3}\,\left(x_{\mathrm{qd}}-x_{\mathrm{qdd}}\right)}{x_{l}-x_{\mathrm{qd}}}\right)}{x_{\mathrm{qdd}}}-\frac{\psi _{q,\mathrm{SG},D,3}\,\left(\frac{\psi _{\mathrm{1d},\mathrm{SG},D,3}\,\left(x_{\mathrm{dd}}-x_{\mathrm{ddd}}\right)}{x_{\mathrm{dd}}-x_{l}}-\psi _{d,\mathrm{SG},D,3}+\frac{\psi _{\mathrm{fd},\mathrm{SG},D,3}\,\left(x_{\mathrm{ddd}}-x_{l}\right)}{x_{\mathrm{dd}}-x_{l}}\right)}{x_{\mathrm{ddd}}}$
      | Automatically generated on 2025-11-01 08:50:30 .
  State_psi_d_SG_D_3_193a7 : Inport
  State_psi_gq_SG_D_3_6ebde : Inport  Port=2
  State_psi_kq_SG_D_3_8ca03 : Inport  Port=3
  State_psi_q_SG_D_3_a96b5 : Inport  Port=4
  State_psi_q_SG_D_3_acbca : Inport  Port=5
  State_psi_1d_SG_D_3_57116 : Inport  Port=6
  State_psi_d_SG_D_3_dbbf4 : Inport  Port=7
  State_psi_fd_SG_D_3_e857c : Inport  Port=8
  Add_24bb6 : Sum
  Add_37085 : Sum
  Add_60ee8 : Sum
  Add_74d45 : Sum
  Add_90d4d : Sum
  Add_d2469 : Sum
  Constant_-1_53aee : Constant  Value=-1
  Constant_-1_b72be : Constant  Value=-1
  Constant_-1_c02ae : Constant  Value=-1
  Constant_-1_f2674 : Constant  Value=-1
  Constant_-1_fc945 : Constant  Value=-1
  Constant_x_dd_195d5 : Constant  Value=x_dd
  Constant_x_dd_2163d : Constant  Value=x_dd
  Constant_x_dd_697d6 : Constant  Value=x_dd
  Constant_x_ddd_119bb : Constant  Value=x_ddd
  Constant_x_ddd_4b7f8 : Constant  Value=x_ddd
  Constant_x_ddd_5d3bb : Constant  Value=x_ddd
  Constant_x_l_05932 : Constant  Value=x_l
  Constant_x_l_1c48d : Constant  Value=x_l
  Constant_x_l_1eb63 : Constant  Value=x_l
  Constant_x_l_294e3 : Constant  Value=x_l
  Constant_x_l_35994 : Constant  Value=x_l
  Constant_x_l_9f7e2 : Constant  Value=x_l
  Constant_x_qd_47b72 : Constant  Value=x_qd
  Constant_x_qd_9a88c : Constant  Value=x_qd
  Constant_x_qd_dc359 : Constant  Value=x_qd
  Constant_x_qdd_371be : Constant  Value=x_qdd
  Constant_x_qdd_5aaff : Constant  Value=x_qdd
  Constant_x_qdd_8ccc9 : Constant  Value=x_qdd
  Divide_03027 : Product  Inputs=*/
  Divide_1eef7 : Product  Inputs=*/
  Divide_7f2e6 : Product  Inputs=*/
  Divide_bee2c : Product  Inputs=*/
  Divide_c5e67 : Product  Inputs=*/
  Divide_f0525 : Product  Inputs=*/
  Product_0a2a6 : Product
  Product_1224f : Product
  Product_18527 : Product
  Product_1fc29 : Product
  Product_2f75e : Product
  Product_3b2c1 : Product
  Product_47f5a : Product
  Product_92125 : Product
  Product_ab470 : Product
  Product_ad394 : Product
  Product_cb38d : Product
  Subtract_1b82e : Sum  Inputs=+-
  Subtract_32d3e : Sum  Inputs=+-
  Subtract_3aedd : Sum  Inputs=+-
  Subtract_9a231 : Sum  Inputs=+-
  Subtract_9a607 : Sum  Inputs=+-
  Subtract_db683 : Sum  Inputs=+-
  Subtract_eebe9 : Sum  Inputs=+-
  Blockout_T_e_SG_D_3_7d8b1 : Outport
  wires:
  State_psi_q_SG_D_3_a96b5/1 -> Add_24bb6/2
  Constant_-1_f2674/1 -> Product_0a2a6/1
  Subtract_9a607/1 -> Product_ad394/2
  State_psi_1d_SG_D_3_57116/1 -> Product_ab470/2
  Constant_-1_c02ae/1 -> Product_3b2c1/1
  Constant_x_l_9f7e2/1 -> Product_3b2c1/2
  Add_74d45/1 -> Subtract_9a607/1
  State_psi_d_SG_D_3_dbbf4/1 -> Add_74d45/2
  Product_3b2c1/1 -> Add_d2469/1
  Constant_x_qdd_371be/1 -> Subtract_eebe9/2
  Add_24bb6/1 -> Product_92125/2
  Constant_x_qdd_8ccc9/1 -> Add_d2469/2
  State_psi_q_SG_D_3_acbca/1 -> Product_ad394/1
  Constant_x_l_1eb63/1 -> Product_0a2a6/2
  Subtract_9a231/1 -> Divide_7f2e6/2
  Constant_x_l_05932/1 -> Subtract_db683/2
  Constant_x_qd_9a88c/1 -> Subtract_eebe9/1
  Constant_-1_53aee/1 -> Product_18527/1
  Subtract_32d3e/1 -> Divide_1eef7/2
  Constant_x_l_35994/1 -> Product_18527/2
  Product_cb38d/1 -> Divide_1eef7/1
  Constant_-1_b72be/1 -> Product_ab470/1
  Product_ab470/1 -> Product_cb38d/1
  Constant_x_dd_697d6/1 -> Subtract_3aedd/1
  Constant_x_ddd_4b7f8/1 -> Subtract_3aedd/2
  Add_37085/1 -> Blockout_T_e_SG_D_3_7d8b1/1
  State_psi_gq_SG_D_3_6ebde/1 -> Product_47f5a/1
  Product_ad394/1 -> Divide_bee2c/1
  Add_d2469/1 -> Product_47f5a/2
  State_psi_fd_SG_D_3_e857c/1 -> Product_2f75e/1
  Product_0a2a6/1 -> Add_90d4d/1
  Constant_x_qd_47b72/1 -> Add_90d4d/2
  Constant_x_dd_2163d/1 -> Subtract_32d3e/1
  State_psi_kq_SG_D_3_8ca03/1 -> Product_1224f/1
  Constant_x_dd_195d5/1 -> Subtract_9a231/1
  Subtract_eebe9/1 -> Product_1224f/2
  Product_92125/1 -> Divide_f0525/1
  Product_18527/1 -> Add_60ee8/1
  Add_90d4d/1 -> Divide_c5e67/2
  Constant_x_qd_dc359/1 -> Add_60ee8/2
  Subtract_3aedd/1 -> Product_cb38d/2
  Constant_x_l_1c48d/1 -> Subtract_32d3e/2
  Constant_x_ddd_5d3bb/1 -> Subtract_db683/1
  Product_47f5a/1 -> Divide_c5e67/1
  Product_1224f/1 -> Divide_03027/1
  Add_60ee8/1 -> Divide_03027/2
  Constant_x_ddd_119bb/1 -> Divide_bee2c/2
  Subtract_db683/1 -> Product_2f75e/2
  Divide_c5e67/1 -> Subtract_1b82e/1
  Constant_x_l_294e3/1 -> Subtract_9a231/2
  Divide_03027/1 -> Subtract_1b82e/2
  Divide_1eef7/1 -> Add_74d45/1
  Product_2f75e/1 -> Divide_7f2e6/1
  Constant_-1_fc945/1 -> Product_1fc29/1
  State_psi_d_SG_D_3_193a7/1 -> Product_1fc29/2
  Subtract_1b82e/1 -> Add_24bb6/1
  Divide_7f2e6/1 -> Subtract_9a607/2
  Product_1fc29/1 -> Product_92125/1
  Constant_x_qdd_5aaff/1 -> Divide_f0525/2
  Divide_f0525/1 -> Add_37085/1
  Divide_bee2c/1 -> Add_37085/2

== system IEEE9_case/SG_D_3/d_E_fd_SG_D_3_block ==
  note: d_E_fd_SG_D_3 in IEEE9_case
      | $\frac{V_{f,\mathrm{SG},D,3}-E_{\mathrm{fd},\mathrm{SG},D,3}\,K_{E}}{T_{E}}$
      | Automatically generated on 2025-11-01 08:50:13 .
  State_E_fd_SG_D_3_4edb4 : Inport
  State_V_f_SG_D_3_2efed : Inport  Port=2
  Add_dd4f8 : Sum
  Constant_-1_3f797 : Constant  Value=-1
  Constant_K_E_e6ee5 : Constant  Value=K_E
  Constant_T_E_1a01d : Constant  Value=T_E
  Divide_ca5c1 : Product  Inputs=*/
  Product_6a3c9 : Product
  Product_bed3b : Product
  Blockout_d_E_fd_SG_D_3_49225 : Outport
  wires:
  State_V_f_SG_D_3_2efed/1 -> Add_dd4f8/2
  Constant_-1_3f797/1 -> Product_bed3b/1
  State_E_fd_SG_D_3_4edb4/1 -> Product_bed3b/2
  Constant_T_E_1a01d/1 -> Divide_ca5c1/2
  Product_bed3b/1 -> Product_6a3c9/1
  Product_6a3c9/1 -> Add_dd4f8/1
  Constant_K_E_e6ee5/1 -> Product_6a3c9/2
  Divide_ca5c1/1 -> Blockout_d_E_fd_SG_D_3_49225/1
  Add_dd4f8/1 -> Divide_ca5c1/1

== system IEEE9_case/SG_D_3/d_Px_1_SG_D_3_block ==
  note: d_Px_1_SG_D_3 in IEEE9_case
      | $\frac{w_{\mathrm{SG},D,3}-2\,\pi \,f_{0}}{T_{w}}-\frac{\mathrm{Px}_{1,\mathrm{SG},D,3}}{T_{w}}$
      | Automatically generated on 2025-11-01 08:50:15 .
  State_Px_1_SG_D_3_67f42 : Inport
  State_w_SG_D_3_88dc5 : Inport  Port=2
  Add_0a644 : Sum
  Add_a163d : Sum
  Constant_-1_269c4 : Constant  Value=-1
  Constant_-2.0_1c4c8 : Constant  Value=-2.0
  Constant_T_w_31684 : Constant  Value=T_w
  Constant_T_w_e126d : Constant  Value=T_w
  Constant_f0_37576 : Constant  Value=f0
  Constant_pi_08385 : Constant  Value=pi
  Divide_4ddd7 : Product  Inputs=*/
  Divide_93e04 : Product  Inputs=*/
  Product_5b68e : Product
  Product_b3285 : Product
  Product_de39e : Product
  Blockout_d_Px_1_SG_D_3_7cdee : Outport
  wires:
  Constant_f0_37576/1 -> Product_de39e/2
  Constant_-1_269c4/1 -> Product_b3285/1
  Constant_-2.0_1c4c8/1 -> Product_5b68e/1
  Constant_pi_08385/1 -> Product_5b68e/2
  Product_5b68e/1 -> Product_de39e/1
  State_w_SG_D_3_88dc5/1 -> Add_0a644/2
  Divide_4ddd7/1 -> Add_a163d/1
  State_Px_1_SG_D_3_67f42/1 -> Product_b3285/2
  Product_de39e/1 -> Add_0a644/1
  Product_b3285/1 -> Divide_4ddd7/1
  Constant_T_w_31684/1 -> Divide_4ddd7/2
  Add_0a644/1 -> Divide_93e04/1
  Constant_T_w_e126d/1 -> Divide_93e04/2
  Divide_93e04/1 -> Add_a163d/2
  Add_a163d/1 -> Blockout_d_Px_1_SG_D_3_7cdee/1

== system IEEE9_case/SG_D_3/d_Px_2_SG_D_3_block ==
  note: d_Px_2_SG_D_3 in IEEE9_case
      | $\frac{\mathrm{Px}_{1,\mathrm{SG},D,3}-T_{2}\,\left(\frac{\mathrm{Px}_{1,\mathrm{SG},D,3}}{T_{w}}-\frac{w_{\mathrm{SG},D,3}-2\,\pi \,f_{0}}{T_{w}}\right)}{T_{1}}-\frac{\mathrm{Px}_{2,\mathrm{SG},D,3}}{T_{1}}$
      | Automatically generated on 2025-11-01 08:50:16 .
  State_Px_2_SG_D_3_ac8d1 : Inport
  State_Px_1_SG_D_3_30b70 : Inport  Port=2
  State_Px_1_SG_D_3_0e345 : Inport  Port=3
  State_w_SG_D_3_fe91f : Inport  Port=4
  Add_2a249 : Sum
  Add_9581a : Sum
  Add_c754d : Sum
  Add_cbb94 : Sum
  Constant_-1_8424b : Constant  Value=-1
  Constant_-1_9681a : Constant  Value=-1
  Constant_-2.0_0026a : Constant  Value=-2.0
  Constant_T_1_b5726 : Constant  Value=T_1
  Constant_T_1_fe63e : Constant  Value=T_1
  Constant_T_2_3c177 : Constant  Value=T_2
  Constant_T_w_93a1f : Constant  Value=T_w
  Constant_T_w_c37f9 : Constant  Value=T_w
  Constant_f0_a6058 : Constant  Value=f0
  Constant_pi_e4f33 : Constant  Value=pi
  Divide_2d581 : Product  Inputs=*/
  Divide_663fb : Product  Inputs=*/
  Divide_d731d : Product  Inputs=*/
  Divide_ee410 : Product  Inputs=*/
  Product_007e2 : Product
  Product_018ef : Product
  Product_1b0b1 : Product
  Product_b9eba : Product
  Product_e1072 : Product
  Blockout_d_Px_2_SG_D_3_e1b1c : Outport
  wires:
  State_Px_1_SG_D_3_0e345/1 -> Product_007e2/2
  Constant_-2.0_0026a/1 -> Product_018ef/1
  Constant_f0_a6058/1 -> Product_e1072/2
  Constant_pi_e4f33/1 -> Product_018ef/2
  Product_018ef/1 -> Product_e1072/1
  State_w_SG_D_3_fe91f/1 -> Add_9581a/2
  Constant_-1_8424b/1 -> Product_007e2/1
  Product_e1072/1 -> Add_9581a/1
  Product_007e2/1 -> Divide_ee410/1
  Constant_T_w_93a1f/1 -> Divide_ee410/2
  Add_9581a/1 -> Divide_2d581/1
  Constant_T_w_c37f9/1 -> Divide_2d581/2
  Divide_ee410/1 -> Add_c754d/1
  Divide_2d581/1 -> Add_c754d/2
  Constant_T_2_3c177/1 -> Product_b9eba/1
  Add_c754d/1 -> Product_b9eba/2
  Constant_-1_9681a/1 -> Product_1b0b1/1
  Product_b9eba/1 -> Add_cbb94/2
  State_Px_2_SG_D_3_ac8d1/1 -> Product_1b0b1/2
  State_Px_1_SG_D_3_30b70/1 -> Add_cbb94/1
  Product_1b0b1/1 -> Divide_d731d/1
  Add_2a249/1 -> Blockout_d_Px_2_SG_D_3_e1b1c/1
  Constant_T_1_b5726/1 -> Divide_d731d/2
  Add_cbb94/1 -> Divide_663fb/1
  Constant_T_1_fe63e/1 -> Divide_663fb/2
  Divide_d731d/1 -> Add_2a249/1
  Divide_663fb/1 -> Add_2a249/2

== system IEEE9_case/SG_D_3/d_Px_3_SG_D_3_block ==
  note: d_Px_3_SG_D_3 in IEEE9_case
      | $\frac{\mathrm{Px}_{2,\mathrm{SG},D,3}+T_{4}\,\left(\frac{\mathrm{Px}_{1,\mathrm{SG},D,3}-T_{2}\,\left(\frac{\mathrm{Px}_{1,\mathrm{SG},D,3}}{T_{w}}-\frac{w_{\mathrm{SG},D,3}-2\,\pi \,f_{0}}{T_{w}}\right)}{T_{1}}-\frac{\mathrm{Px}_{2,\mathrm{SG},D,3}}{T_{1}}\right)}{T_{3}}-\frac{\mathrm{Px}_{3,\mathrm{SG},D,3}}{T_{3}}$
      | Automatically generated on 2025-11-01 08:50:19 .
  State_Px_3_SG_D_3_8aa31 : Inport
  State_Px_2_SG_D_3_c6c25 : Inport  Port=2
  State_Px_2_SG_D_3_7d1eb : Inport  Port=3
  State_Px_1_SG_D_3_a37cd : Inport  Port=4
  State_Px_1_SG_D_3_f96ae : Inport  Port=5
  State_w_SG_D_3_532bc : Inport  Port=6
  Add_26123 : Sum
  Add_3956e : Sum
  Add_80b49 : Sum
  Add_850f0 : Sum
  Add_85fae : Sum
  Add_fb20b : Sum
  Constant_-1_33820 : Constant  Value=-1
  Constant_-1_ba278 : Constant  Value=-1
  Constant_-1_d9ac4 : Constant  Value=-1
  Constant_-2.0_28b95 : Constant  Value=-2.0
  Constant_T_1_49d6f : Constant  Value=T_1
  Constant_T_1_bc9f8 : Constant  Value=T_1
  Constant_T_2_183e1 : Constant  Value=T_2
  Constant_T_3_41ef3 : Constant  Value=T_3
  Constant_T_3_daed8 : Constant  Value=T_3
  Constant_T_4_2f4b5 : Constant  Value=T_4
  Constant_T_w_88d62 : Constant  Value=T_w
  Constant_T_w_95695 : Constant  Value=T_w
  Constant_f0_13e3e : Constant  Value=f0
  Constant_pi_f5a8d : Constant  Value=pi
  Divide_30f7a : Product  Inputs=*/
  Divide_37129 : Product  Inputs=*/
  Divide_792f1 : Product  Inputs=*/
  Divide_8a1fe : Product  Inputs=*/
  Divide_8f26c : Product  Inputs=*/
  Divide_c708d : Product  Inputs=*/
  Product_0ea77 : Product
  Product_1337f : Product
  Product_3cfd2 : Product
  Product_639bb : Product
  Product_b5bb1 : Product
  Product_c4009 : Product
  Product_efd78 : Product
  Blockout_d_Px_3_SG_D_3_549f5 : Outport
  wires:
  State_Px_1_SG_D_3_f96ae/1 -> Product_3cfd2/2
  Constant_f0_13e3e/1 -> Product_639bb/2
  Constant_-2.0_28b95/1 -> Product_efd78/1
  Add_85fae/1 -> Divide_8f26c/1
  Constant_pi_f5a8d/1 -> Product_efd78/2
  Product_efd78/1 -> Product_639bb/1
  State_w_SG_D_3_532bc/1 -> Add_fb20b/2
  Constant_T_w_95695/1 -> Divide_30f7a/2
  Constant_-1_33820/1 -> Product_3cfd2/1
  Product_639bb/1 -> Add_fb20b/1
  Product_3cfd2/1 -> Divide_30f7a/1
  Add_fb20b/1 -> Divide_c708d/1
  Product_c4009/1 -> Divide_37129/1
  Constant_T_w_88d62/1 -> Divide_c708d/2
  Divide_30f7a/1 -> Add_26123/1
  Divide_c708d/1 -> Add_26123/2
  Constant_T_2_183e1/1 -> Product_0ea77/1
  Add_26123/1 -> Product_0ea77/2
  Constant_-1_ba278/1 -> Product_c4009/1
  State_Px_2_SG_D_3_7d1eb/1 -> Product_c4009/2
  State_Px_1_SG_D_3_a37cd/1 -> Add_85fae/1
  Constant_T_3_41ef3/1 -> Divide_792f1/2
  Product_0ea77/1 -> Add_85fae/2
  Constant_T_1_bc9f8/1 -> Divide_37129/2
  Add_80b49/1 -> Product_1337f/2
  Constant_T_1_49d6f/1 -> Divide_8f26c/2
  Divide_8a1fe/1 -> Add_850f0/2
  Divide_37129/1 -> Add_80b49/1
  Divide_8f26c/1 -> Add_80b49/2
  Constant_T_4_2f4b5/1 -> Product_1337f/1
  Constant_-1_d9ac4/1 -> Product_b5bb1/1
  State_Px_3_SG_D_3_8aa31/1 -> Product_b5bb1/2
  State_Px_2_SG_D_3_c6c25/1 -> Add_3956e/1
  Product_1337f/1 -> Add_3956e/2
  Product_b5bb1/1 -> Divide_792f1/1
  Add_3956e/1 -> Divide_8a1fe/1
  Constant_T_3_daed8/1 -> Divide_8a1fe/2
  Divide_792f1/1 -> Add_850f0/1
  Add_850f0/1 -> Blockout_d_Px_3_SG_D_3_549f5/1
